simulink model "chap1_11"  (R2023b)
settings: Solver=ode5  StartTime=0.0  StopTime=1  FixedStep=0.001  RelTol=1e-3  EnableMultiTasking=on
settings Model: Creator=CorgiQvm  LastModifiedBy=CorgiQvm
settings DataIOCC: LimitDataPoints=on  ReturnWorkspaceOutputs=off
settings ModelReferenceCC: PropagateSignalLabelsOutOfModel=off

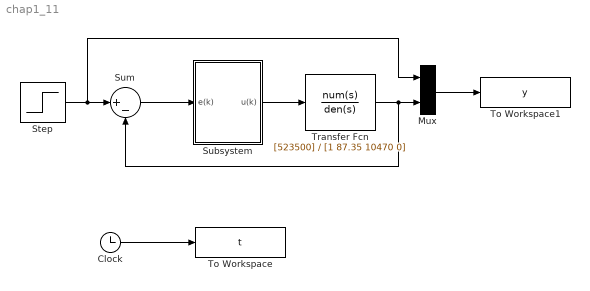
== system chap1_11 ==
  Clock : Clock
  Mux : Mux  Inputs=2
  Step : Step  Time=0  SampleTime=0
  Subsystem : Subsystem  mask{Kp=0.5, Ki=0.001, Kd=0.001, T=0.001, U_m=10}
      mask prompts: Kp "Proportional Kp"; Ki "Integrator Ki"; Kd "Derivative Kd"; T "Sampling period T"; U_m "Actuator Limit"
      mask DialogControl ParameterGroupVar Prompt: 参数
      mask Display: disp('Discrete PID');
  Sum : Sum  Inputs=|+-  SaturateOnIntegerOverflow=on
  To Workspace : ToWorkspace  VariableName=t  SampleTime=-1
  To Workspace1 : ToWorkspace  VariableName=y  SampleTime=-1
  Transfer Fcn : TransferFcn  Numerator=[523500]  Denominator=[1 87.35 10470 0]
  wires:
  Mux/1 -> To Workspace1/1
  Transfer Fcn/1 -> Sum/2, Mux/2
  Subsystem/1(u(k)) -> Transfer Fcn/1
  Sum/1 -> Subsystem/1(e(k))
  Step/1 -> Mux/1, Sum/1
  Clock/1 -> To Workspace/1

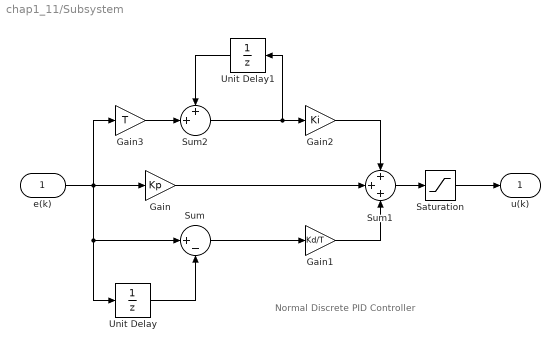
== system chap1_11/Subsystem ==
  note: Normal Discrete PID Controller
  e(k) : Inport
  Gain : Gain  Gain=Kp  SaturateOnIntegerOverflow=on  OutDataTypeStr=Inherit: Same as input  ParamDataTypeStr=Inherit: Same as input
  Gain1 : Gain  Gain=Kd/T  SaturateOnIntegerOverflow=on  OutDataTypeStr=Inherit: Same as input  ParamDataTypeStr=Inherit: Same as input
  Gain2 : Gain  Gain=Ki  SaturateOnIntegerOverflow=on  OutDataTypeStr=Inherit: Same as input  ParamDataTypeStr=Inherit: Same as input
  Gain3 : Gain  Gain=T  SaturateOnIntegerOverflow=on  OutDataTypeStr=Inherit: Same as input  ParamDataTypeStr=Inherit: Same as input
  Saturation : Saturate  UpperLimit=U_m  LowerLimit=-U_m
  Sum : Sum  Inputs=|+-  SaturateOnIntegerOverflow=on
  Sum1 : Sum  Inputs=+++  SaturateOnIntegerOverflow=on
  Sum2 : Sum  Inputs=++|  SaturateOnIntegerOverflow=on
  Unit Delay : UnitDelay  SampleTime=-1  HasFrameUpgradeWarning=on
  Unit Delay1 : UnitDelay  SampleTime=-1  HasFrameUpgradeWarning=on
  u(k) : Outport
  wires:
  Saturation/1 -> u(k)/1
  e(k)/1 -> Gain3/1, Unit Delay/1, Sum/1, Gain/1
  Sum2/1 -> Unit Delay1/1, Gain2/1
  Gain3/1 -> Sum2/2
  Gain/1 -> Sum1/2
  Unit Delay/1 -> Sum/2
  Sum1/1 -> Saturation/1
  Gain2/1 -> Sum1/1
  Unit Delay1/1 -> Sum2/1
  Gain1/1 -> Sum1/3
  Sum/1 -> Gain1/1
